simulink model "ammclib_amclib_field_weakening_s32k11x"  (Simulink 9.0)
settings: Solver=FixedStepDiscrete  StartTime=0.0  StopTime=10  FixedStep=0.001  RelTol=1e-3  EnableMultiTasking=on
InitFcn:
  | mbd_s32k_consistency_checks(bdroot(gcs));
undefined symbols (not defined in the file or in its folder): LQFP, thumb
libraries: ammclib_bam_s32k11x x4, simulink x3, mbd_s32k1xx_ec_toolbox x2
Description:
  | This model tests the AMMCLIB AMCLIB Field Weakening blocks
  | 
  | Validation:
  | - Run the model in Simulation and compare the Inputs vs Outputs results.
  | - Open Freemaster (ammclib_amclib_field_weakening_s32k11x.pmp) and compare the HW results against the Simulated ones
settings Model: Creator=NXP MBDT Team  LastModifiedBy=nxf35172
settings DataIOCC: ExternalInput=off  InitialState=off  LimitDataPoints=on  SaveOutput=off  SignalLogging=off  SaveTime=off
settings OptimizationCC: DefaultParameterBehavior=Inlined  LifeSpan=1
settings DebuggingCC: SolverPrmCheckMsg=warning  InheritedTsInSrcMsg=none  SingleTaskRateTransMsg=error  ParameterPrecisionLossMsg=none  UnconnectedInputMsg=error  UnconnectedOutputMsg=error  UnconnectedLineMsg=error  AllowSymbolicDim=off  UnknownTsInhSupMsg=error  StateNameClashWarn=warning
settings HardwareCC: ProdLargestAtomicInteger=Long  ProdLargestAtomicFloat=Double  ProdEndianess=LittleEndian  ProdHWDeviceType=ARM Compatible->ARM Cortex
settings SFSimCC: MATLABDynamicMemAlloc=off
settings RTWCC: SystemTargetFile=mbd_s32k.tlc  MakeCommand=mbd_s32k_make_rtw COPY_MDLREF_INCLUDES=0  TemplateMakefile=mbd_s32k.tmf  Description=Model Based Design Toolbox S32K14x Code Generation Target
settings CodeAppCC: IgnoreCustomStorageClasses=off
settings STFCustomTargetCC: CombineOutputUpdateFcns=on  ERTCustomFileBanners=on  SupportContinuousTime=off  SupportNonInlinedSFcns=off  RemoveResetFunc=on  MATLABClassNameForMDSCustomization=Simulink.SoftwareTarget.ERTCustomization  GRTInterface=off  SystemTargetFile=mbd_s32k14.tlc
settings ERTTargetCC: MultiwordLength=2048  ParMdlRefBuildCompliant=off  CompOptLevelCompliant=off  ConcurrentExecutionCompliant=off  ModelStepFunctionPrototypeControlCompliant=off  CPPClassGenCompliant=off  UseToolchainInfoCompliant=off  InlinedParameterPlacement=NonHierarchical  ERTCustomFileTemplate=example_file_process.tlc  ConvertIfToSwitch=off  SuppressUnreachableDefaultCases=off

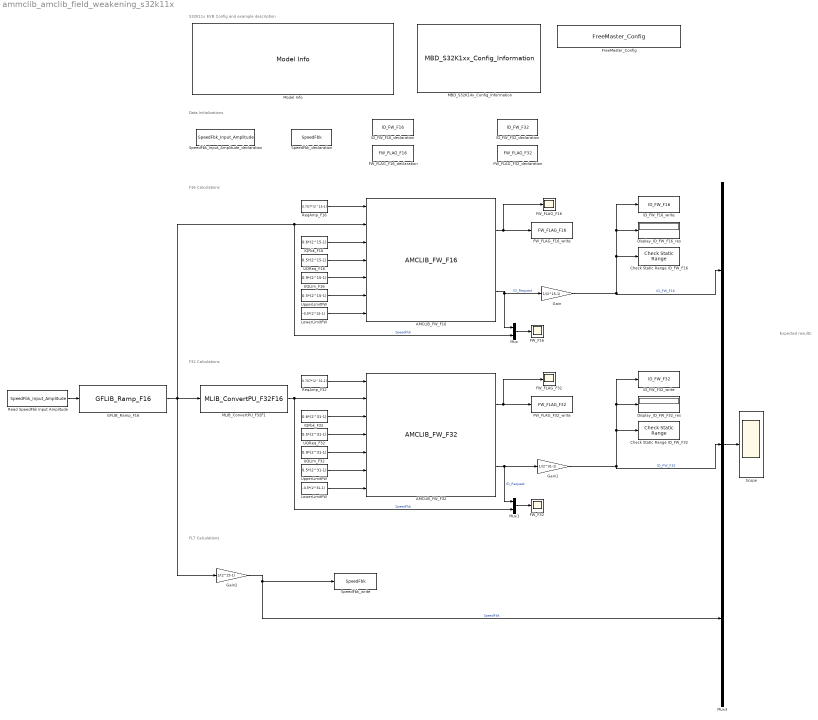
== system ammclib_amclib_field_weakening_s32k11x ==
  note: Expected results:
  note: S32K11x EVB Config and example description
  note: Data Initializations
  note: F16 Calculations
  note: F32 Calculations
  note: FLT Calculations
  AMCLIB_FW_F16 : ammclib_bam_s32k11x/AMCLIB/bam_f16/AMCLIB_FW_F16  u16NSamplesFW=3  f16PropGainFW=0.001*(2^15-1)  s16PropGainShiftFW=0  f16IntegGainFW=0.0001*(2^15-1)  s16IntegGainShiftFW=0
  AMCLIB_FW_F32 : ammclib_bam_s32k11x/AMCLIB/bam_f32/AMCLIB_FW_F32  u16NSamplesFW=3  f32PropGainFW=0.001*(2^31-1)  s16PropGainShiftFW=0  f32IntegGainFW=0.0001*(2^31-1)  s16IntegGainShiftFW=0
  "Check Static Range ID_FW_F16 " : simulink/Model Verification/Check  Static Range  Description=0 <= u <= 0.707*(2^15-1)  max=0.707*(2^15-1)  max_included=on  min=0  min_included=on  enabled=on  stopWhenAssertionFail=on  export=off  icon=graphic
      settings: SourceProductName=Simulink  SourceProductBaseCode=SL
  "Check Static Range ID_FW_F32 " : simulink/Model Verification/Check  Static Range  Description=0 <= u <= 0.707*(2^31-1)  max=0.707*(2^31-1)  max_included=on  min=0  min_included=on  enabled=on  stopWhenAssertionFail=on  export=off  icon=graphic
      settings: SourceProductName=Simulink  SourceProductBaseCode=SL
  Display_ID_FW_F16_res : Display
  Display_ID_FW_F32_res : Display
  FW_F16 : Scope
  FW_F32 : Scope
  FW_FLAG_F16 : Scope
  FW_FLAG_F16_declaration : DataStoreMemory  Priority=3  DataStoreName=FW_FLAG_F16  ReadBeforeWriteMsg=warning  WriteAfterWriteMsg=warning  WriteAfterReadMsg=warning  ShowAdditionalParam=off  OutDataTypeStr=uint16
  FW_FLAG_F16_write : DataStoreWrite  DataStoreName=FW_FLAG_F16
  FW_FLAG_F32 : Scope
  FW_FLAG_F32_declaration : DataStoreMemory  Priority=3  DataStoreName=FW_FLAG_F32  ReadBeforeWriteMsg=warning  WriteAfterWriteMsg=warning  WriteAfterReadMsg=warning  ShowAdditionalParam=off  OutDataTypeStr=uint16
  FW_FLAG_F32_write : DataStoreWrite  DataStoreName=FW_FLAG_F32
  FreeMaster_Config : mbd_s32k1xx_ec_toolbox/Utility Blocks/FreeMaster_Config  interface=LPUART0  baudrate=19200  rxd=PTB0: [LPUART0_RX | Receive]  txd=PTB1: [LPUART0_TX | Transmit]  mode=Short Interrupt  isr_prio=1  show_adv_opts=on  use_scope=on  max_scope_vars=8  use_recorder=on  max_rec_vars=8  rec_buff_size=1024  rec_timebase=0 milliseconds  comm_buffer_size_auto=on  comm_buffer_size=255  comm_rqueue_size_default=on  comm_rqueue_size=32
  GFLIB_Ramp_F16 : ammclib_bam_s32k11x/GFLIB/bam_f16/GFLIB_Ramp_F16  f16RampUp=2  f16RampDown=2
  Gain : Gain  Gain=1/(2^15-1)  OutDataTypeStr=Inherit: Inherit via back propagation
  Gain1 : Gain  Gain=1/(2^31-1)  OutDataTypeStr=Inherit: Inherit via back propagation
  Gain2 : Gain  Gain=1/(2^15-1)  OutDataTypeStr=Inherit: Inherit via back propagation
  ID_FW_F16_declaration : DataStoreMemory  Priority=2  DataStoreName=ID_FW_F16  ReadBeforeWriteMsg=warning  WriteAfterWriteMsg=warning  WriteAfterReadMsg=warning  ShowAdditionalParam=off  OutDataTypeStr=single
  ID_FW_F16_write : DataStoreWrite  DataStoreName=ID_FW_F16
  ID_FW_F32_declaration : DataStoreMemory  Priority=2  DataStoreName=ID_FW_F32  ReadBeforeWriteMsg=warning  WriteAfterWriteMsg=warning  WriteAfterReadMsg=warning  ShowAdditionalParam=off  OutDataTypeStr=single
  ID_FW_F32_write : DataStoreWrite  DataStoreName=ID_FW_F32
  IQFbk_F16 : Constant  Value=0.6*(2^15-1)  OutDataTypeStr=Inherit: Inherit via back propagation
  IQFbk_F32 : Constant  Value=0.6*(2^31-1)  OutDataTypeStr=Inherit: Inherit via back propagation
  LowerLimitFW : Constant  Value=-0.5*(2^15-1)  OutDataTypeStr=Inherit: Inherit via back propagation
  "LowerLimitFW " : Constant  Value=-0.5*(2^31-1)  OutDataTypeStr=Inherit: Inherit via back propagation
  MBD_S32K14x_Config_Information : mbd_s32k1xx_ec_toolbox/MBD_S32K1xx_Config_Information  Priority=0  mbdt_ver=0  disp_str=|  config_params=[]  mcu_target_name=S32K116  mcu_target_package=48-LQFP  mcu_target_sram_size=17KB  mcu_system_clock_freq=40  mcu_xtal_freq=External 40  mcu_steptick_timer=LPIT Channel 0  mcu_steptick_prio=0  ds_import_enable=on  target_compiler=GCC  target_memory=FLASH  gcc_target_compile_opts=-mcpu=cortex-m0plus -mthumb -O1 -g -gstrict-dwarf  gcc_target_assemble_opts=-mcpu=cortex-m0plus -mthumb -g  gcc_target_link_opts=-mcpu=cortex-m0plus -mthumb  gcc_target_default_lcf=on  gcc_target_user_lcf=S32K116_17_flash.ld  ghs_target_compile_opts=-mcpu=cortexm0plus -mthumb -fsoft -Ogeneral -Wundef -Wimplicit-int -Wshadow -Wtrigraphs --no_commons --gnu_asm -gnu99 -gdwarf-2 -G  ghs_target_assemble_opts=-mcpu=cortexm0plus -mthumb -fsoft --gnu_asm  ghs_target_link_opts=-mcpu=cortexm0plus -mthumb -fsoft  ghs_target_default_lcf=off  ghs_target_user_lcf=S32K116_17_flash.ld  iar_target_compile_opts=--thumb -Ol -e --debug --dlib_config normal  iar_target_assemble_opts=--thumb  iar_target_link_opts=--no_exceptions --vfe --inline  iar_target_default_lcf=off  iar_target_user_lcf=S32K116_17_flash.icf  pil_download_enable=off  rbl_download_enable=on  rbl_start_delay=5000000  rbl_download_interface=OpenSDA  rbl_restart_request=off  rbl_com_port=Custom  rbl_com_port_custom=COM1  pil_download_rate=57600  pil_opensda_drive=Custom  pil_opensda_drive_custom=D  pil_uart_instance=0  pil_uart_rx=PTA2: [LPUART0_RX | Receive]  pil_uart_tx=PTA3: [LPUART0_TX | Transmit]  FTM_PWM_PcrCheckEnDis=on  FTM_Input_Edge_Inputs_PcrCheckEnDis=on  FTM_Dual_Edge_Inputs_PcrCheckEnDis=on  FTM_Quadrature_Inputs_PcrCheckEnDis=on  FTM_Hall_Sensor_Inputs_PcrCheckEnDis=on  LPTMR_PcrCheckEnDis=on  PIT_PcrCheckEnDis=on  RTC_PcrCheckEnDis=on  FlexCAN_PcrCheckEnDis=on  LIN_PcrCheckEnDis=on  FlexIO_PcrCheckEnDis=on  LPI2C_PcrCheckEnDis=on  LPSPI_PcrCheckEnDis=on  LPUART_PcrCheckEnDis=on  CMP_PcrCheckEnDis=on  GPIO_OutputPcrCheckEnDis=on  GPIO_InputPcrCheckEnDis=on  SBC_PcrCheckEnDis=on  AMMCLIB_PcrCheckEnDis=on  FM_PcrCheckEnDis=on  Profile_PcrCheckEnDis=on  ConfigParams_PcrCheckEnDis=on  ModelRef_PcrCheckEnDis=on  PDB0_PcrCheckEnDis=on  CSEc_PcrCheckEnDis=on  eDMA_PcrCheckEnDis=on  ADC_PcrCheckEnDis=on  WDOG_PcrCheckEnDis=on
      | Target : S32K142-16KB_SRAM
      | Package : 100-pin
      | System clock : 80 MHz
      | XTAL clock : External 8 MHz
      | Compiler : GCC
      | Target Type : FLASH
      | Download Code after build : (OpenSDA: E)
      | Step Tick Interrupt Priority : 15
  MLIB_ConvertPU_F32F1 : ammclib_bam_s32k11x/MLIB/bam_f32/MLIB_ConvertPU_F32F16
  Model Info : simulink/Model-Wide Utilities/Model Info  Frame=off  DisplayStringWithTags=|  HorizontalTextAlignment=Left  LeftAlignmentValue=0.02
      | Model Name: %<ModelName>
      | 
      | Description: %<Description>
  Mux : Mux  Inputs=2
  Mux1 : Mux  Inputs=2
  Mux3 : Mux  Inputs=3
  Read SpeedFbk Input Amplitude : DataStoreRead  DataStoreName=SpeedFbk_Input_Amplitude
  ReqAmp_F16 : Constant  Value=0.707*(2^15-1)  OutDataTypeStr=Inherit: Inherit via back propagation
  ReqAmp_F32 : Constant  Value=0.707*(2^31-1)  OutDataTypeStr=Inherit: Inherit via back propagation
  Scope : Scope
  SpeedFbk_Input_Amplitude_declaration : DataStoreMemory  Priority=1  DataStoreName=SpeedFbk_Input_Amplitude  WriteAfterWriteMsg=warning  WriteAfterReadMsg=warning  InitialValue=0.25*(2^15-1)  ShowAdditionalParam=off  OutMin=-32768  OutMax=32767  OutDataTypeStr=int16
  SpeedFbk_declaration : DataStoreMemory  Priority=1  DataStoreName=SpeedFbk  WriteAfterWriteMsg=warning  WriteAfterReadMsg=warning  ShowAdditionalParam=off  OutMin=-1  OutMax=1  OutDataTypeStr=single
  SpeedFbk_write : DataStoreWrite  DataStoreName=SpeedFbk
  UQLim_F16 : Constant  Value=0.9*(2^15-1)  OutDataTypeStr=Inherit: Inherit via back propagation
  UQLim_F32 : Constant  Value=0.9*(2^31-1)  OutDataTypeStr=Inherit: Inherit via back propagation
  UQReq_F16 : Constant  Value=0.5*(2^15-1)  OutDataTypeStr=Inherit: Inherit via back propagation
  UQReq_F32 : Constant  Value=0.5*(2^31-1)  OutDataTypeStr=Inherit: Inherit via back propagation
  UpperLimitFW : Constant  Value=0.5*(2^15-1)  OutDataTypeStr=Inherit: Inherit via back propagation
  "UpperLimitFW " : Constant  Value=0.5*(2^31-1)  OutDataTypeStr=Inherit: Inherit via back propagation
  wires:
  UpperLimitFW/1 -> AMCLIB_FW_F16/6
  LowerLimitFW/1 -> AMCLIB_FW_F16/7
  AMCLIB_FW_F16/1 -> FW_FLAG_F16/1, FW_FLAG_F16_write/1
  Read SpeedFbk Input Amplitude/1 -> GFLIB_Ramp_F16/1
  ReqAmp_F16/1 -> AMCLIB_FW_F16/1
  AMCLIB_FW_F16/2 -> Mux/1, Gain/1  "ID_Request"
  Gain/1 -> Mux3/1, "Check Static Range ID_FW_F16 "/1, ID_FW_F16_write/1, Display_ID_FW_F16_res/1  "ID_FW_F16"
  Mux/1 -> FW_F16/1
  Mux3/1 -> Scope/1
  GFLIB_Ramp_F16/1 -> Gain2/1, Mux/2, AMCLIB_FW_F16/2, MLIB_ConvertPU_F32F1/1  "SpeedFbk"
  IQFbk_F16/1 -> AMCLIB_FW_F16/3
  UQLim_F16/1 -> AMCLIB_FW_F16/5
  UQReq_F16/1 -> AMCLIB_FW_F16/4
  "UpperLimitFW "/1 -> AMCLIB_FW_F32/6
  "LowerLimitFW "/1 -> AMCLIB_FW_F32/7
  AMCLIB_FW_F32/1 -> FW_FLAG_F32/1, FW_FLAG_F32_write/1
  ReqAmp_F32/1 -> AMCLIB_FW_F32/1
  AMCLIB_FW_F32/2 -> Gain1/1, Mux1/1  "ID_Request"
  Gain1/1 -> Mux3/2, Display_ID_FW_F32_res/1, ID_FW_F32_write/1, "Check Static Range ID_FW_F32 "/1  "ID_FW_F32"
  Mux1/1 -> FW_F32/1
  MLIB_ConvertPU_F32F1/1 -> Mux1/2, AMCLIB_FW_F32/2  "SpeedFbk"
  IQFbk_F32/1 -> AMCLIB_FW_F32/3
  UQLim_F32/1 -> AMCLIB_FW_F32/5
  UQReq_F32/1 -> AMCLIB_FW_F32/4
  Gain2/1 -> Mux3/3, SpeedFbk_write/1  "SpeedFbk"
